simulink model "PM_fnc22_Xregen_Detection_TestHarness1"  (R2022a)
settings: Solver=FixedStepDiscrete  StartTime=0  StopTime=65.0009  FixedStep=0.01  RelTol=1e-3
values from neighbouring files (symbols this model uses):
  rate_ms = 10    [PM_fnc1000_tc01_iter01_testsignal_builder.m]    (also in PM_fnc21_tc01_iter01_testsignal_builder.m; PM_fnc22_tc01_iter01_testsignal_builder.m)
settings Model: Creator=306427  LastModifiedBy=306427
settings SolverCC: ZeroCrossAlgorithm=Adaptive

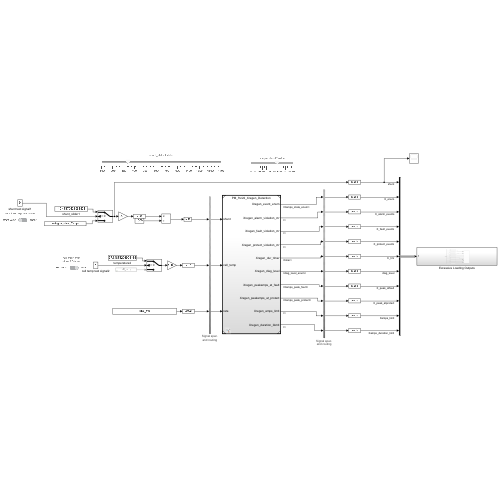
[thumbnail: Simulink's stored preview of the top-level diagram]
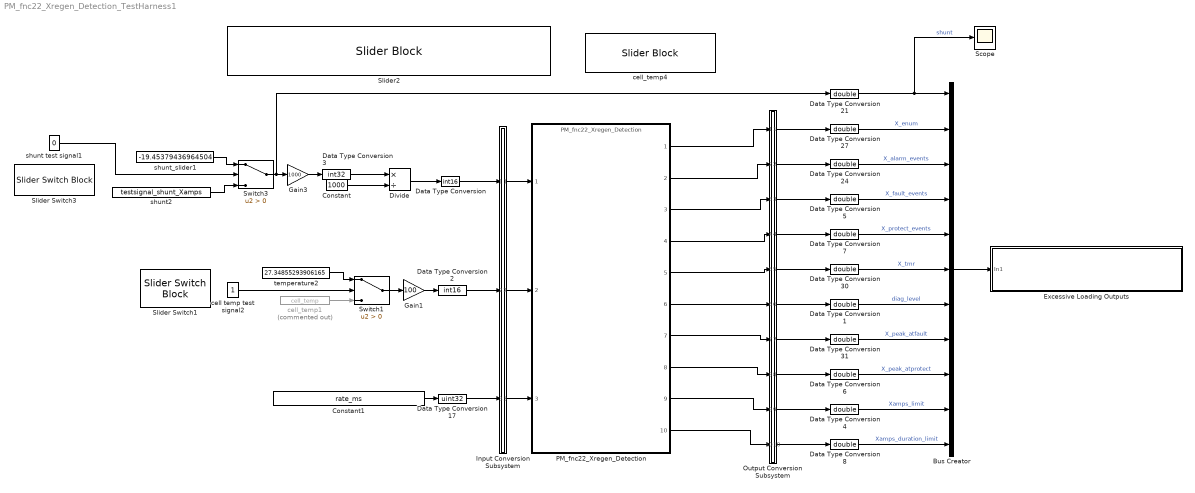
== system PM_fnc22_Xregen_Detection_TestHarness1 ==
  Bus Creator : BusCreator  Inputs=11
  Constant : Constant  Value=1000
  Constant1 : Constant  Value=rate_ms
  Data Type Conversion : DataTypeConversion  OutDataTypeStr=int16  SaturateOnIntegerOverflow=off  RndMeth=Floor
  Data Type Conversion{1,4..8,21,24,27,30..31} (11 alike) : DataTypeConversion  OutDataTypeStr=double  SaturateOnIntegerOverflow=off  RndMeth=Floor
  Data Type Conversion17 : DataTypeConversion  OutDataTypeStr=uint32  SaturateOnIntegerOverflow=off  RndMeth=Floor
  Data Type Conversion2 : DataTypeConversion  OutDataTypeStr=int16  SaturateOnIntegerOverflow=off  RndMeth=Floor
  Data Type Conversion3 : DataTypeConversion  OutDataTypeStr=int32  SaturateOnIntegerOverflow=off  RndMeth=Floor
  Divide : Product  Inputs=*/  OutDataTypeStr=int32  SaturateOnIntegerOverflow=on
  Excessive Loading Outputs : Subsystem
  Gain1 : Gain  Gain=100
  Gain3 : Gain  Gain=1000
  Input Conversion Subsystem : Subsystem  Tag=__SLT_ICS__  Description=|
      | Signal spec.
      | and routing
      settings: AttributesFormatString=%<Description>
  Output Conversion Subsystem : Subsystem  Tag=__SLT_OCS__  Description=|
      | Signal spec.
      | and routing
      settings: AttributesFormatString=%<Description>
  PM_fnc22_Xregen_Detection : ModelReference  ModelNameDialog=PM_fnc22_Xregen_Detection  SimulationMode=Normal  ModelReferenceVersion=1.30
  Scope : Scope
  Slider Switch1 : SliderSwitchBlock
      settings: Values={{'from wksp', 'slider'}, [0 1]}
  Slider Switch3 : SliderSwitchBlock
      settings: Values={{'from wksp', 'slider'}, [0 1]}
  Slider2 : SliderBlock  ScaleMin=-500  ScaleMax=+1700
  Switch1 : Switch  Criteria=u2 > Threshold  SaturateOnIntegerOverflow=off  InputSameDT=off
  Switch3 : Switch  Criteria=u2 > Threshold  SaturateOnIntegerOverflow=off  InputSameDT=off
  cell temp test signal2 : Constant
  cell_temp1 : FromWorkspace  Commented=on  VariableName=cell_temp  OutDataTypeStr=double  SampleTime=[0, 1]
  cell_temp4 : SliderBlock  ScaleMin=-40  ScaleMax=70
  shunt test signal1 : Constant  Value=0
  shunt2 : FromWorkspace  VariableName=testsignal_shunt_Xamps  OutDataTypeStr=double
  shunt_slider1 : Constant  Value=-19.45379436964504  OutDataTypeStr=double
  temperature2 : Constant  Value=27.34855293906165  OutDataTypeStr=double
  wires:
  Data Type Conversion/1 -> Input Conversion Subsystem/1(Inport_1)
  Data Type Conversion2/1 -> Input Conversion Subsystem/2(Inport_2)
  Output Conversion Subsystem/8(Outport_8) -> Data Type Conversion6/1
  Output Conversion Subsystem/5(Outport_5) -> Data Type Conversion30/1
  Output Conversion Subsystem/3(Outport_3) -> Data Type Conversion5/1
  shunt_slider1/1 -> Switch3/1
  Data Type Conversion6/1 -> Bus Creator/9  "X_peak_atprotect"
  Gain3/1 -> Data Type Conversion3/1
  Constant/1 -> Divide/2
  cell temp test signal2/1 -> Switch1/2
  Output Conversion Subsystem/9(Outport_9) -> Data Type Conversion4/1
  Gain1/1 -> Data Type Conversion2/1
  Data Type Conversion31/1 -> Bus Creator/8  "X_peak_atfault"
  Output Conversion Subsystem/1(Outport_1) -> Data Type Conversion27/1
  Data Type Conversion21/1 -> Scope/1, Bus Creator/1  "shunt"
  Data Type Conversion17/1 -> Input Conversion Subsystem/3(Inport_3)
  Data Type Conversion7/1 -> Bus Creator/5  "X_protect_events"
  Data Type Conversion30/1 -> Bus Creator/6  "X_tmr"
  Output Conversion Subsystem/4(Outport_4) -> Data Type Conversion7/1
  cell_temp1/1 -> Switch1/3
  Switch3/1 -> Data Type Conversion21/1, Gain3/1
  Data Type Conversion4/1 -> Bus Creator/10  "Xamps_limit"
  Output Conversion Subsystem/6(Outport_6) -> Data Type Conversion1/1
  temperature2/1 -> Switch1/1
  shunt test signal1/1 -> Switch3/2
  Output Conversion Subsystem/10(Outport_10) -> Data Type Conversion8/1
  Data Type Conversion1/1 -> Bus Creator/7  "diag_level"
  Output Conversion Subsystem/2(Outport_2) -> Data Type Conversion24/1
  Data Type Conversion27/1 -> Bus Creator/2  "X_enum"
  Output Conversion Subsystem/7(Outport_7) -> Data Type Conversion31/1
  Constant1/1 -> Data Type Conversion17/1
  shunt2/1 -> Switch3/3
  Data Type Conversion5/1 -> Bus Creator/4  "X_fault_events"
  Data Type Conversion24/1 -> Bus Creator/3  "X_alarm_events"
  Bus Creator/1 -> Excessive Loading Outputs/1(In1)
  Data Type Conversion3/1 -> Divide/1
  Switch1/1 -> Gain1/1
  Data Type Conversion8/1 -> Bus Creator/11  "Xamps_duration_limit"
  Divide/1 -> Data Type Conversion/1
  PM_fnc22_Xregen_Detection/1 -> Output Conversion Subsystem/1(Inport_1)
  PM_fnc22_Xregen_Detection/2 -> Output Conversion Subsystem/2(Inport_2)
  PM_fnc22_Xregen_Detection/3 -> Output Conversion Subsystem/3(Inport_3)
  PM_fnc22_Xregen_Detection/4 -> Output Conversion Subsystem/4(Inport_4)
  PM_fnc22_Xregen_Detection/5 -> Output Conversion Subsystem/5(Inport_5)
  PM_fnc22_Xregen_Detection/6 -> Output Conversion Subsystem/6(Inport_6)
  PM_fnc22_Xregen_Detection/7 -> Output Conversion Subsystem/7(Inport_7)
  PM_fnc22_Xregen_Detection/8 -> Output Conversion Subsystem/8(Inport_8)
  PM_fnc22_Xregen_Detection/9 -> Output Conversion Subsystem/9(Inport_9)
  PM_fnc22_Xregen_Detection/10 -> Output Conversion Subsystem/10(Inport_10)
  Input Conversion Subsystem/1(Outport_1) -> PM_fnc22_Xregen_Detection/1
  Input Conversion Subsystem/2(Outport_2) -> PM_fnc22_Xregen_Detection/2
  Input Conversion Subsystem/3(Outport_3) -> PM_fnc22_Xregen_Detection/3

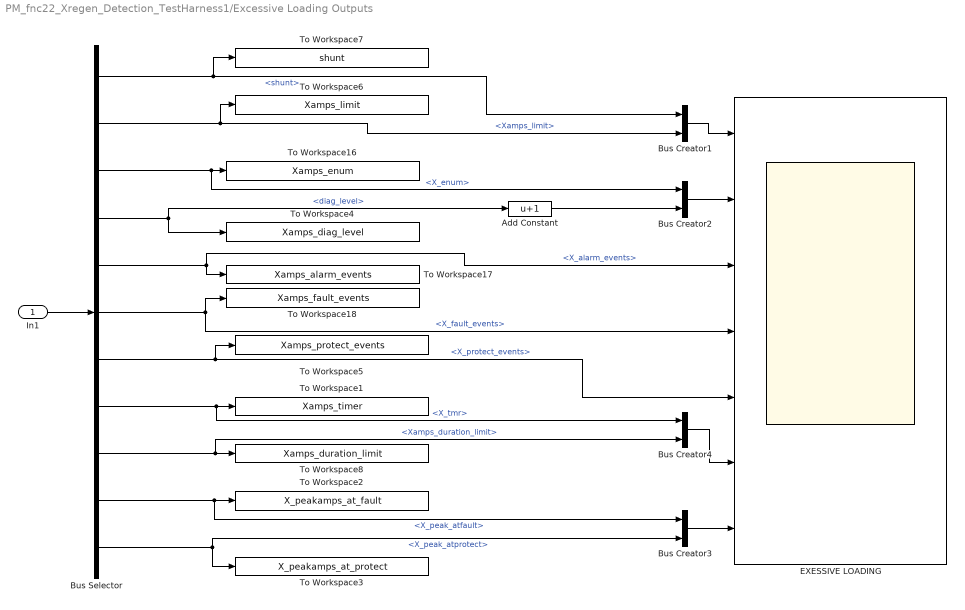
== system PM_fnc22_Xregen_Detection_TestHarness1/Excessive Loading Outputs ==
  In1 : Inport
  Add Constant : Bias  Bias=1  SaturateOnIntegerOverflow=off
  Bus Creator{1..4} (4 alike) : BusCreator  Inputs=2
  Bus Selector : BusSelector  OutputSignals=shunt,Xamps_limit,X_enum,diag_level,X_alarm_events,X_fault_events,X_protect_events,X_tmr,Xamps_duration_limit,X_peak_atfault,X_peak_atprotect
  EXESSIVE LOADING : Scope  NumInputPorts=7
  To Workspace1 : ToWorkspace  VariableName=Xamps_timer  SampleTime=-1
      settings: Save2DSignal=2-D array (concatenate along first dimension)
  To Workspace16 : ToWorkspace  VariableName=Xamps_enum  SampleTime=-1
      settings: Save2DSignal=2-D array (concatenate along first dimension)
  To Workspace17 : ToWorkspace  VariableName=Xamps_alarm_events  SampleTime=-1
      settings: Save2DSignal=2-D array (concatenate along first dimension)
  To Workspace18 : ToWorkspace  VariableName=Xamps_fault_events  SampleTime=-1
      settings: Save2DSignal=2-D array (concatenate along first dimension)
  To Workspace2 : ToWorkspace  VariableName=X_peakamps_at_fault  SampleTime=-1
      settings: Save2DSignal=2-D array (concatenate along first dimension)
  To Workspace3 : ToWorkspace  VariableName=X_peakamps_at_protect  SampleTime=-1
      settings: Save2DSignal=2-D array (concatenate along first dimension)
  To Workspace4 : ToWorkspace  VariableName=Xamps_diag_level  SampleTime=-1
      settings: Save2DSignal=2-D array (concatenate along first dimension)
  To Workspace5 : ToWorkspace  VariableName=Xamps_protect_events  SampleTime=-1
      settings: Save2DSignal=2-D array (concatenate along first dimension)
  To Workspace6 : ToWorkspace  VariableName=Xamps_limit  SampleTime=-1
      settings: Save2DSignal=2-D array (concatenate along first dimension)
  To Workspace7 : ToWorkspace  VariableName=shunt  SampleTime=-1
      settings: Save2DSignal=2-D array (concatenate along first dimension)
  To Workspace8 : ToWorkspace  VariableName=Xamps_duration_limit  SampleTime=-1
      settings: Save2DSignal=2-D array (concatenate along first dimension)
  wires:
  In1/1 -> Bus Selector/1
  Bus Selector/3 -> Bus Creator2/1, To Workspace16/1  "<X_enum>"
  Bus Selector/5 -> EXESSIVE LOADING/3, To Workspace17/1  "<X_alarm_events>"
  Bus Creator1/1 -> EXESSIVE LOADING/1
  Bus Selector/1 -> To Workspace7/1, Bus Creator1/1  "<shunt>"
  Bus Selector/6 -> To Workspace18/1, EXESSIVE LOADING/4  "<X_fault_events>"
  Bus Selector/8 -> Bus Creator4/1, To Workspace1/1  "<X_tmr>"
  Bus Selector/10 -> To Workspace2/1, Bus Creator3/1  "<X_peak_atfault>"
  Bus Selector/2 -> To Workspace6/1, Bus Creator1/2  "<Xamps_limit>"
  Bus Selector/4 -> Add Constant/1, To Workspace4/1  "<diag_level>"
  Bus Selector/11 -> To Workspace3/1, Bus Creator3/2  "<X_peak_atprotect>"
  Bus Selector/7 -> To Workspace5/1, EXESSIVE LOADING/5  "<X_protect_events>"
  Bus Creator2/1 -> EXESSIVE LOADING/2
  Bus Creator3/1 -> EXESSIVE LOADING/7
  Add Constant/1 -> Bus Creator2/2
  Bus Selector/9 -> To Workspace8/1, Bus Creator4/2  "<Xamps_duration_limit>"
  Bus Creator4/1 -> EXESSIVE LOADING/6

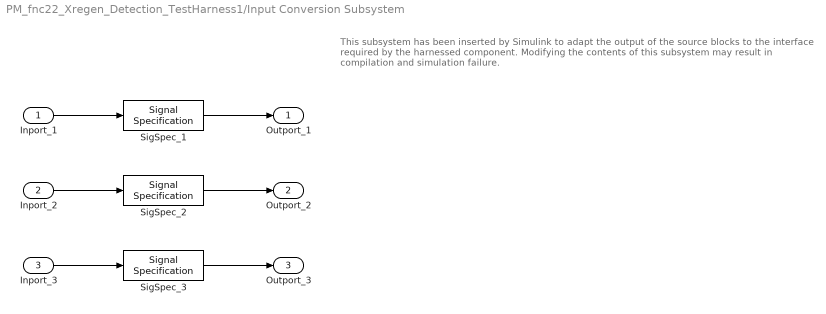
== system PM_fnc22_Xregen_Detection_TestHarness1/Input Conversion Subsystem ==
  note: This subsystem has been inserted by Simulink to adapt the output of the source blocks to the interface required by the harnessed component.
      |  Modifying the contents of this subsystem may result in compilation and simulation failure.
  Inport_1 : Inport
  Inport_2 : Inport  Port=2
  Inport_3 : Inport  Port=3
  SigSpec_1 : SignalSpecification  OutDataTypeStr=int16  Dimensions=[1]  SampleTime=0.01
  SigSpec_2 : SignalSpecification  OutDataTypeStr=int16  Dimensions=[1]  SampleTime=0.01
  SigSpec_3 : SignalSpecification  OutDataTypeStr=uint32  Dimensions=[1]  SampleTime=0.01
  Outport_1 : Outport
  Outport_2 : Outport  Port=2
  Outport_3 : Outport  Port=3
  wires:
  SigSpec_1/1 -> Outport_1/1
  Inport_1/1 -> SigSpec_1/1
  SigSpec_2/1 -> Outport_2/1
  Inport_2/1 -> SigSpec_2/1
  SigSpec_3/1 -> Outport_3/1
  Inport_3/1 -> SigSpec_3/1

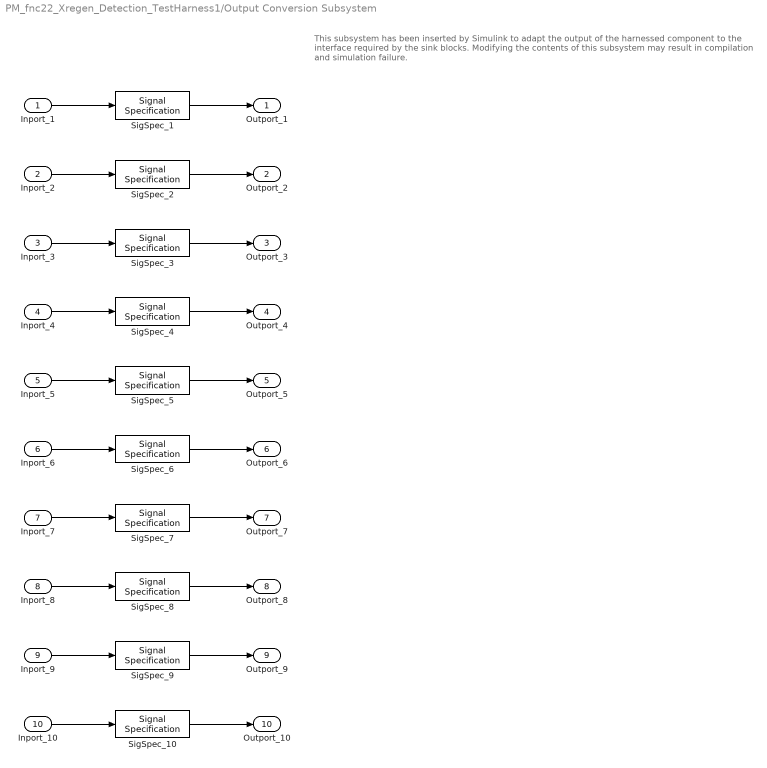
== system PM_fnc22_Xregen_Detection_TestHarness1/Output Conversion Subsystem ==
  note: This subsystem has been inserted by Simulink to adapt the output of the harnessed component to the interface required by the sink blocks.
      |  Modifying the contents of this subsystem may result in compilation and simulation failure.
  Inport_1 : Inport
  Inport_2 : Inport  Port=2
  Inport_3 : Inport  Port=3
  Inport_4 : Inport  Port=4
  Inport_5 : Inport  Port=5
  Inport_6 : Inport  Port=6
  Inport_7 : Inport  Port=7
  Inport_8 : Inport  Port=8
  Inport_9 : Inport  Port=9
  Inport_10 : Inport  Port=10
  SigSpec_1 : SignalSpecification  OutDataTypeStr=uint8  Dimensions=[1]  SampleTime=0.01
  SigSpec_{3..5,10} (4 alike) : SignalSpecification  OutDataTypeStr=uint16  Dimensions=[1]  SampleTime=0.01
  SigSpec_2 : SignalSpecification  OutDataTypeStr=uint32  Dimensions=[1]  SampleTime=0.01
  SigSpec_6 : SignalSpecification  OutDataTypeStr=uint8  Dimensions=[1]  SampleTime=0.01
  SigSpec_7 : SignalSpecification  OutDataTypeStr=int16  Dimensions=[1]  SampleTime=0.01
  SigSpec_8 : SignalSpecification  OutDataTypeStr=int16  Dimensions=[1]  SampleTime=0.01
  SigSpec_9 : SignalSpecification  OutDataTypeStr=int16  Dimensions=[1]  SampleTime=0.01
  Outport_1 : Outport
  Outport_2 : Outport  Port=2
  Outport_3 : Outport  Port=3
  Outport_4 : Outport  Port=4
  Outport_5 : Outport  Port=5
  Outport_6 : Outport  Port=6
  Outport_7 : Outport  Port=7
  Outport_8 : Outport  Port=8
  Outport_9 : Outport  Port=9
  Outport_10 : Outport  Port=10
  wires:
  Inport_1/1 -> SigSpec_1/1
  SigSpec_1/1 -> Outport_1/1
  Inport_2/1 -> SigSpec_2/1
  SigSpec_2/1 -> Outport_2/1
  Inport_3/1 -> SigSpec_3/1
  SigSpec_3/1 -> Outport_3/1
  Inport_4/1 -> SigSpec_4/1
  SigSpec_4/1 -> Outport_4/1
  Inport_5/1 -> SigSpec_5/1
  SigSpec_5/1 -> Outport_5/1
  Inport_6/1 -> SigSpec_6/1
  SigSpec_6/1 -> Outport_6/1
  Inport_7/1 -> SigSpec_7/1
  SigSpec_7/1 -> Outport_7/1
  Inport_8/1 -> SigSpec_8/1
  SigSpec_8/1 -> Outport_8/1
  Inport_9/1 -> SigSpec_9/1
  SigSpec_9/1 -> Outport_9/1
  Inport_10/1 -> SigSpec_10/1
  SigSpec_10/1 -> Outport_10/1
